simulink model "nadir_pointing"  (R2021a)
settings: Solver=VariableStepAuto  StartTime=0.0  StopTime=1.5*Torb  RelTol=1e-3
libraries: sharedtransform x2
settings Model: Creator=Laura  LastModifiedBy=Laura
settings SolverCC: ZeroCrossAlgorithm=Adaptive
settings DebuggingCC: IgnoredZcDiagnostic=none

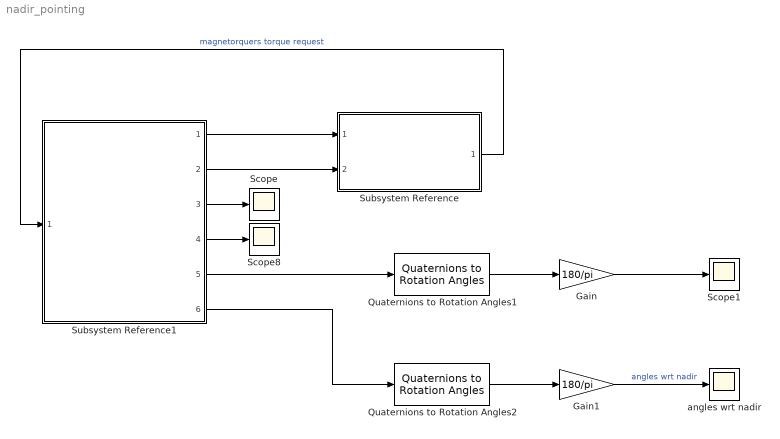
== system nadir_pointing ==
  Gain : Gain  Gain=180/pi
  Gain1 : Gain  Gain=180/pi
  Quaternions to Rotation Angles1 : sharedtransform/Quaternions to Rotation Angles  rotationOrder=ZYX  aMode=aMode
      settings: SourceProductBaseCode=AE,PW,DR,MT,UV,VE
  Quaternions to Rotation Angles2 : sharedtransform/Quaternions to Rotation Angles  rotationOrder=ZYX  aMode=aMode
      settings: SourceProductBaseCode=AE,PW,DR,MT,UV,VE
  Scope : Scope
  Scope1 : Scope
  Scope8 : Scope
  Subsystem Reference : Subsystem  ReferencedSubsystem=PD_roll
  Subsystem Reference1 : Subsystem  ReferencedSubsystem=DKE_detumbling
  angles wrt nadir : Scope
  wires:
  Quaternions to Rotation Angles2/1 -> Gain1/1
  Subsystem Reference1/5 -> Quaternions to Rotation Angles1/1
  Subsystem Reference/1 -> Subsystem Reference1/1  "magnetorquers torque request"
  Subsystem Reference1/6 -> Quaternions to Rotation Angles2/1
  Subsystem Reference1/3 -> Scope/1
  Quaternions to Rotation Angles1/1 -> Gain/1
  Subsystem Reference1/4 -> Scope8/1
  Subsystem Reference1/2 -> Subsystem Reference/2
  Subsystem Reference1/1 -> Subsystem Reference/1
  Gain1/1 -> angles wrt nadir/1  "angles wrt nadir"
  Gain/1 -> Scope1/1
